simulink model "animationtest"  (R2016a)
settings: Solver=VariableStepAuto  StartTime=0.0  StopTime=100  RelTol=1e-3
libraries: vrlib x2, simulink x2
settings Model: Creator=VAIO  LastModifiedBy=VAIO

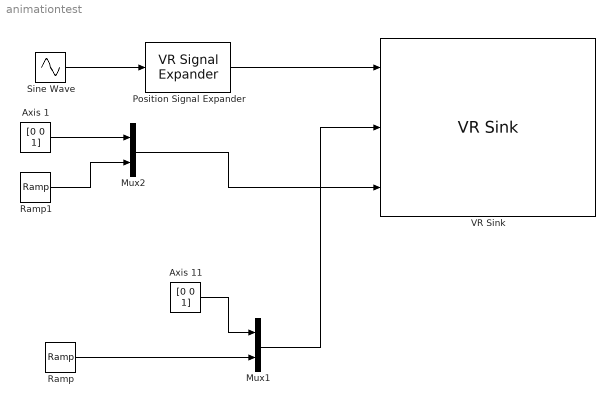
== system animationtest ==
  Axis 1 : Constant  Value=[0 0 1]
  Axis 11 : Constant  Value=[0 0 1]
  Mux1 : Mux  Inputs=2
  Mux2 : Mux  Inputs=2
  Position Signal Expander : vrlib/VR Signal Expander  outwidth=3  outidx=[1]
  Ramp : simulink/Sources/Ramp  slope=-0.8  start=0  X0=0
  Ramp1 : simulink/Sources/Ramp  slope=1  start=0  X0=0
  Sine Wave : Sin  SampleTime=0
  VR Sink : vrlib/VR Sink  InstantiateOnLoad=on  SampleTime=0.06  ViewEnable=on  RemoteChange=off  RemoteView=off  FieldsWritten=Cart.translation.3.1.1.double#Joint1.rotation.4.1.1.double#joint2.rotation.4.1.1.double  WorldFileName=Pendulum159.wrl  AutoView=off  VideoDimensions=[]  AllowVariableSize=off  FigureProperties="{'Position', 'Name', 'Viewpoint', 'CameraBound', 'CameraDirection', 'CameraPosition', 'CameraUpVector', 'ZoomFactor', 'Antialiasing', 'Headlight', 'Lighting', 'NavPanel', 'Sound', 'StatusBar', 'Stereo3D', 'Stereo3DCameraOffset', 'Stereo3DHIT', 'ToolBar', 'Textures', 'Transparency', 'Triad', 'Wireframe', 'NavZones', 'NavMode', 'NavSpeed', 'CaptureFileFormat', 'CaptureFileName', 'Record2DCompressMethod', 'Record2DCompressQuality', 'Record2D', 'Record2DFileName', 'Record2DFPS'; [6.6900000000000000e+02   1.7900000000000000e+02   5.7600000000000000e+02   3.5000000000000000e+02], '', '', 'on', [0.0000000000000000e+00   0.0000000000000000e+00  -1.0000000000000000e+00], [0.0000000000000000e+00   0.0000000000000000e+00   1.0000000000000000e+01], [0.0000000000000000e+00   1.0000000000000000e+00   0.0000000000000000e+00], [1.0000000000000000e+00], 'on', 'on', 'on', 'halfbar', 'on', 'on', 'off', [1.0000000149011612e-01], [0.0000000000000000e+00], 'on', 'on', 'on', 'none', 'off', 'off', 'fly', 'normal', 'tif', '%f_anim_%n.tif', 'auto', [7.5000000000000000e+01], 'off', '%f_anim_%n.avi', 'auto'}"
  wires:
  Mux1/1 -> VR Sink/2
  Ramp/1 -> Mux1/2
  Axis 11/1 -> Mux1/1
  Axis 1/1 -> Mux2/1
  Ramp1/1 -> Mux2/2
  Mux2/1 -> VR Sink/3
  Sine Wave/1 -> Position Signal Expander/1
  Position Signal Expander/1 -> VR Sink/1
